simulink model "Roll"  (R2020a)
settings: Solver=ode3  StartTime=0.0  StopTime=inf  FixedStep=0.02  RelTol=1e-3  EnableMultiTasking=on
libraries: simulink_extras x1, arduinolib x1
settings Model: SILPILModeSetting=veronly  ExtModeTrigDuration=2  Creator=Ali  LastModifiedBy=Ali
settings OptimizationCC: EnhancedBackFolding=on  PassReuseOutputArgsAs=Individual arguments  ZeroExternalMemoryAtStartup=off  ZeroInternalMemoryAtStartup=off  MaxStackSize=64  OptimizeBlockOrder=speed  DifferentSizesBufferReuse=on  OptimizationCustomize=off  EfficientTunableParamExpr=on
settings DebuggingCC: ParameterTunabilityLossMsg=error
settings HardwareCC: ProdBitPerInt=16  ProdBitPerPointer=16  ProdBitPerSizeT=16  ProdBitPerPtrDiffT=16  ProdLargestAtomicFloat=None  ProdWordSize=8  ProdHWDeviceType=Atmel->AVR
settings SFSimCC: MATLABDynamicMemAlloc=off
settings RTWCC: SystemTargetFile=ert.tlc  HardwareBoard=Arduino Mega 2560  TLCOptions=-aInlineSetEventsForThisBaseRateFcn=TLC_FALSE -aSuppressMultiTaskScheduler=TLC_FALSE -aRateBasedStepFcn=1  TemplateMakefile=ert_default_tmf  Toolchain=Arduino AVR  BuildConfiguration=Faster Runs
settings CodeAppCC: ForceParamTrailComments=on  IgnoreCustomStorageClasses=off  OperatorAnnotations=on  SimulinkDataObjDesc=on  SFDataObjDesc=on  InsertBlockDesc=on
settings ERTTargetCC: SupportContinuousTime=on  SupportVariableSizeSignals=on  ExtModeStaticAllocSize=2048

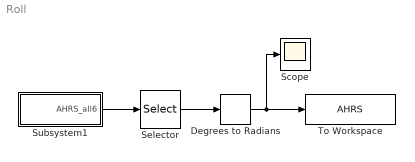
== system Roll ==
  Degrees to Radians : simulink_extras/Transformations/Degrees to Radians
  Scope : Scope
  Selector : Selector  InputPortWidth=6  IndexOptions=Index vector (dialog)  Indices=[1 4]  OutputSizes=1
  Subsystem1 : Subsystem
  To Workspace : ToWorkspace  VariableName=AHRS  SampleTime=-1
  wires:
  Subsystem1/1(AHRS_all6) -> Selector/1
  Selector/1 -> Degrees to Radians/1
  Degrees to Radians/1 -> Scope/1, To Workspace/1

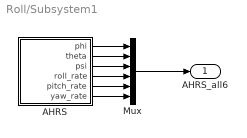
== system Roll/Subsystem1 ==
  AHRS : Subsystem
  Mux : Mux  Inputs=6
  AHRS_all6 : Outport
  wires:
  Mux/1 -> AHRS_all6/1
  AHRS/1(phi) -> Mux/1
  AHRS/5(pitch_rate) -> Mux/5
  AHRS/2(theta) -> Mux/2
  AHRS/4(roll_rate) -> Mux/4
  AHRS/3(psi) -> Mux/3
  AHRS/6(yaw_rate) -> Mux/6

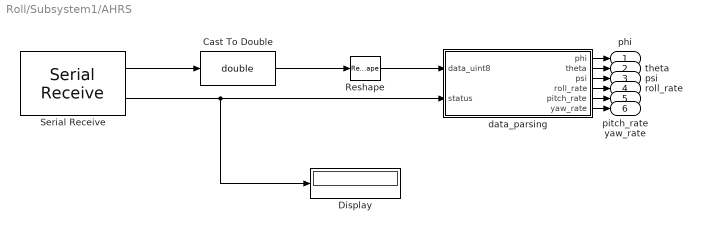
== system Roll/Subsystem1/AHRS ==
  Cast To Double : DataTypeConversion  OutDataTypeStr=double
  Display : Display
  Reshape : Reshape
  Serial Receive : arduinolib/Serial Receive  isARMArch=off  portNumber=1  DataType=uint8  Datalength=32  SampleTime=0.02  showOutStatus=on  blockPlatform=arduino
      settings: SourceProductBaseCode=ARDUINO
  data_parsing : MATLAB Function  TreatAsAtomicUnit=on
  phi : Outport
  theta : Outport  Port=2
  psi : Outport  Port=3
  roll_rate : Outport  Port=4
  pitch_rate : Outport  Port=5
  yaw_rate : Outport  Port=6
  wires:
  data_parsing/2(theta) -> theta/1
  data_parsing/3(psi) -> psi/1
  data_parsing/4(roll_rate) -> roll_rate/1
  Reshape/1 -> data_parsing/1(data_uint8)
  data_parsing/1(phi) -> phi/1
  data_parsing/5(pitch_rate) -> pitch_rate/1
  Serial Receive/2 -> Display/1, data_parsing/2(status)
  data_parsing/6(yaw_rate) -> yaw_rate/1
  Cast To Double/1 -> Reshape/1
  Serial Receive/1 -> Cast To Double/1

== matlab function Roll/Subsystem1/AHRS/data_parsing ==
  data: phi output size=1; data_uint8 input size=32; theta output size=1; psi output size=1; roll_rate output size=1; pitch_rate output size=1; yaw_rate output size=1; status input
function [phi,theta,psi,roll_rate,pitch_rate,yaw_rate] = fcn(data_uint8, status)
persistent stepp check_sum...
    phi_p theta_p psi_p roll_rate_p pitch_rate_p yaw_rate_p...
    phi_last theta_last psi_last roll_rate_last pitch_rate_last yaw_rate_last;
%% Initialize
if isempty(stepp)
    stepp=0;
    check_sum=0;
    phi_p=0;
    theta_p=0;
    psi_p=0;
    roll_rate_p=0;
    pitch_rate_p=0;
    yaw_rate_p=0;
    phi_last=0;
    theta_last=0;
    psi_last=0;
    roll_rate_last=0;
    pitch_rate_last=0;
    yaw_rate_last=0;
end
angle_scale=.0109863;  % 1/91.0222
rate_scale=1/16;
%% Check Each Byte
if status
    for i = 1:length(data_uint8)
        if (data_uint8(i)==115 && stepp==0)
            stepp=1;
            check_sum=data_uint8(i);
        elseif(stepp==1 && data_uint8(i)==110)
            stepp=stepp+1;
            check_sum=check_sum+data_uint8(i);
        elseif(stepp==2 && data_uint8(i)==112)
            stepp=stepp+1;
            check_sum=check_sum+data_uint8(i);
        elseif(stepp==3 && data_uint8(i)==212)
            stepp=stepp+1;
            check_sum=check_sum+data_uint8(i);
        elseif(stepp==4 && data_uint8(i)==112)
            stepp=stepp+1;
            check_sum=check_sum+data_uint8(i);
        elseif(stepp==5)
            phi_p=data_uint8(i)*256;
            stepp=stepp+1;
            check_sum=check_sum+data_uint8(i);
        elseif(stepp==6)
            phi_p=phi_p+data_uint8(i);
            stepp=stepp+1;
            check_sum=check_sum+data_uint8(i);
        elseif(stepp==7)
            theta_p=data_uint8(i)*256;
            stepp=stepp+1;
            check_sum=check_sum+data_uint8(i);
        elseif(stepp==8)
            theta_p=theta_p+data_uint8(i);
            stepp=stepp+1;
            check_sum=check_sum+data_uint8(i);
        elseif(stepp==9)
            psi_p=data_uint8(i)*256;
            stepp=stepp+1;
            check_sum=check_sum+data_uint8(i);
        elseif(stepp==10)
            psi_p=psi_p+data_uint8(i);
            stepp=stepp+1;
            check_sum=check_sum+data_uint8(i);
        elseif(stepp==11 || stepp==12)
            if(data_uint8(i)==0)
                stepp=stepp+1;
            else
                stepp=0;
            end
        elseif(stepp==13)
            roll_rate_p=data_uint8(i)*256;
            stepp=stepp+1;
            check_sum=check_sum+data_uint8(i);
        elseif(stepp==14)
            roll_rate_p=roll_rate_p+data_uint8(i);
            stepp=stepp+1;
            check_sum=check_sum+data_uint8(i);
        elseif(stepp==15)
            pitch_rate_p=data_uint8(i)*256;
            stepp=stepp+1;
            check_sum=check_sum+data_uint8(i);
        elseif(stepp==16)
            pitch_rate_p=pitch_rate_p+data_uint8(i);
            stepp=stepp+1;
            check_sum=check_sum+data_uint8(i);
        elseif(stepp==17)
            yaw_rate_p=data_uint8(i)*256;
            stepp=stepp+1;
            check_sum=check_sum+data_uint8(i);
        elseif(stepp==18)
            yaw_rate_p=yaw_rate_p+data_uint8(i);
            stepp=stepp+1;
            check_sum=check_sum+data_uint8(i);
        elseif(stepp==19 || stepp==20)
            if(data_uint8(i)==0)
                stepp=stepp+1;
            else
                stepp=0;
            end
        elseif(stepp==21 || stepp==22 || stepp==23 || stepp==24)
            stepp=stepp+1;
            check_sum=check_sum+data_uint8(i);
        elseif(stepp==25)
            if (floor(check_sum/256)==data_uint8(i))
                stepp=stepp+1;
            else
                stepp=0;
            end
        elseif(stepp==26)
            if(mod(check_sum,256)==data_uint8(i))
                phi_last=double(typecast(uint16(phi_p), 'int16'))*angle_scale;
                if mod(phi_last,360)>180
                    phi_last=mod(phi_last,360)-360;
                else
                    phi_last=mod(phi_last,360);
                end
                theta_last=double(typecast(uint16(theta_p), 'int16'))*angle_scale;
                if mod(theta_last,360)>180
                    theta_last=mod(theta_last,360)-360;
                else
                    theta_last=mod(theta_last,360);
                end
                psi_last=double(typecast(uint16(psi_p), 'int16'))*angle_scale;
                if mod(psi_last,360)>180
                    psi_last=mod(psi_last,360)-360;
                else
                    psi_last=mod(psi_last,360);
                end
                roll_rate_last=double(typecast(uint16(roll_rate_p), 'int16'))*rate_scale;
                if mod(roll_rate_last,360)>180
                    roll_rate_last=mod(roll_rate_last,360)-360;
                else
                    roll_rate_last=mod(roll_rate_last,360);
                end
                pitch_rate_last=double(typecast(uint16(pitch_rate_p), 'int16'))*rate_scale;
                if mod(pitch_rate_last,360)>180
                    pitch_rate_last=mod(pitch_rate_last,360)-360;
                else
                    pitch_rate_last=mod(pitch_rate_last,360);
                end
                yaw_rate_last=double(typecast(uint16(yaw_rate_p), 'int16'))*rate_scale;
                if mod(yaw_rate_last,360)>180
                    yaw_rate_last=mod(yaw_rate_last,360)-360;
                else
                    yaw_rate_last=mod(yaw_rate_last,360);
                end
            end
            stepp=0;
        end
    end
end

%% Assign Last True Data to Output
phi=phi_last;
theta=theta_last;
psi=psi_last;
roll_rate=roll_rate_last;
pitch_rate=pitch_rate_last;
yaw_rate=yaw_rate_last;
